simulink model "Quadrotor_Model3D_2018a"  (R2018a)
settings: Solver=VariableStepAuto  StartTime=0.0  StopTime=300  RelTol=1e-3
settings Model: Creator=Slu03  LastModifiedBy=Charles
settings DebuggingCC: LibraryContextMissingDiagnostic=warning
settings SFSimCC: SimUseLocalCustomCode=on
settings RTWCC: RTWUseLocalCustomCode=on

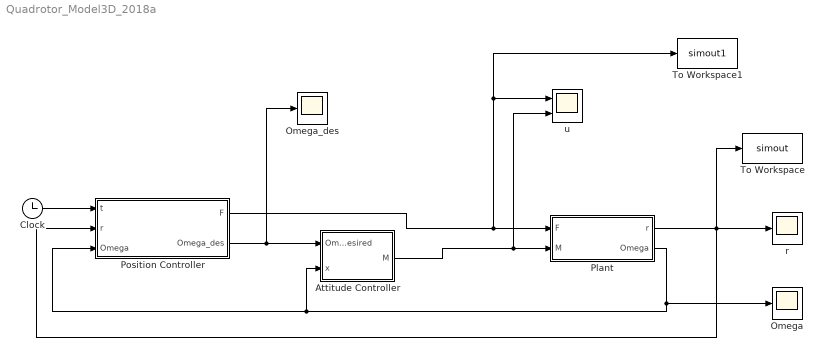
== system Quadrotor_Model3D_2018a ==
  Attitude Controller : MATLAB Function  TreatAsAtomicUnit=on
  Clock : Clock
  Omega : Scope
  Omega_des : Scope
  Plant : Subsystem
  Position Controller : MATLAB Function  TreatAsAtomicUnit=on
  To Workspace : ToWorkspace  VariableName=simout  SaveFormat=Timeseries  SampleTime=-1
  To Workspace1 : ToWorkspace  VariableName=simout1  SaveFormat=Timeseries  SampleTime=-1
  r : Scope
  u : Scope  NumInputPorts=2
  wires:
  Plant/1(r) -> r/1, Position Controller/2(r), To Workspace/1
  Clock/1 -> Position Controller/1(t)
  Position Controller/2(Omega_des) -> Omega_des/1, Attitude Controller/1(Omega_desired)
  Attitude Controller/1(M) -> u/2, Plant/2(M)
  Position Controller/1(F) -> To Workspace1/1, u/1, Plant/1(F)
  Plant/2(Omega) -> Omega/1, Position Controller/3(Omega), Attitude Controller/2(x)

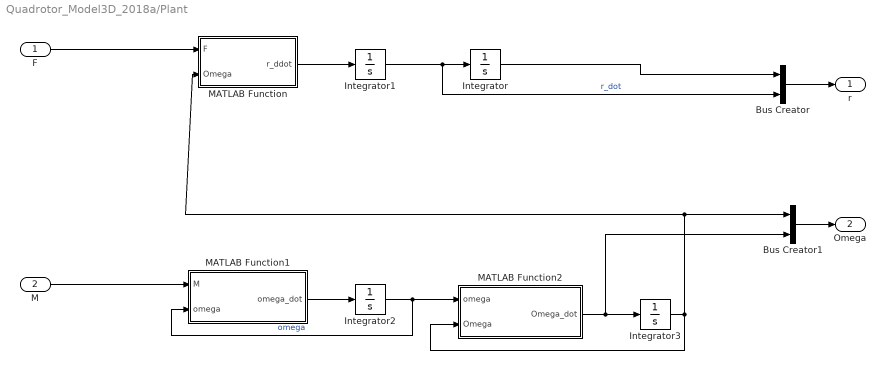
== system Quadrotor_Model3D_2018a/Plant ==
  F : Inport
  M : Inport  Port=2
  Bus Creator : BusCreator  Inputs=2
  Bus Creator1 : BusCreator  Inputs=2
  Integrator : Integrator  InitialCondition=[2,2,0]
  Integrator1 : Integrator
  Integrator2 : Integrator
  Integrator3 : Integrator
  MATLAB Function : MATLAB Function  TreatAsAtomicUnit=on
  MATLAB Function1 : MATLAB Function  TreatAsAtomicUnit=on
  MATLAB Function2 : MATLAB Function  TreatAsAtomicUnit=on
  r : Outport
  Omega : Outport  Port=2
  wires:
  Integrator1/1 -> Bus Creator/2, Integrator/1  "r_dot"
  MATLAB Function/1(r_ddot) -> Integrator1/1
  Integrator2/1 -> MATLAB Function1/2(omega), MATLAB Function2/1(omega)  "omega"
  MATLAB Function1/1(omega_dot) -> Integrator2/1
  MATLAB Function2/1(Omega_dot) -> Bus Creator1/2, Integrator3/1
  Integrator3/1 -> MATLAB Function2/2(Omega), Bus Creator1/1, MATLAB Function/2(Omega)
  F/1 -> MATLAB Function/1(F)
  M/1 -> MATLAB Function1/1(M)
  Bus Creator/1 -> r/1
  Integrator/1 -> Bus Creator/1
  Bus Creator1/1 -> Omega/1

== matlab function Quadrotor_Model3D_2018a/Attitude Controller ==
  data: Omega_desired input; M output; x input
function M = fcn(Omega_desired,x)
kdphi = 20;
kpphi = 100;
kdtheta = 20;
kptheta = 100;
kdpsi = 8;
kppsi = 16;
kd = [kdphi,0,0;0,kdtheta,0;0,0,kdpsi];
kp = [kpphi,0,0;0,kptheta,0;0,0,kppsi];
I = 10^(-5)*[1.43 0 0; 0 1.43 0;0 0 2.89];

Omega_dot = x(4:6);
Omega = x(1:3);
phi = Omega(1);
theta = Omega(2);
psi = Omega(3);

W_inv = [1, 0 ,-sin(theta);0 ,cos(phi),cos(theta)*sin(phi) ; 0 ,-sin(phi),cos(theta)*cos(phi)];
omega = W_inv*Omega_dot;
omega_bracket = [0,-omega(3),omega(2);omega(3),0,-omega(1);-omega(2),omega(1),0];
omega_dot = omega_bracket*I*omega;

M = I*W_inv*(kd*(-Omega_dot)+kp*(Omega_desired-Omega))+omega_dot;

== matlab function Quadrotor_Model3D_2018a/Plant/MATLAB Function ==
  data: F input size=1; Omega input size=3; r_ddot output size=3
function r_ddot = fcn(F,Omega)
g = [0;0;9.8];
m = 0.03;
phi = Omega(1);
theta = Omega(2);
psi = Omega(3);
Rx = [1,0,0; 0,cos(phi),-sin(phi);0,sin(phi),cos(phi)];
Ry = [cos(theta),0,sin(theta);0,1,0;-sin(theta),0,cos(theta)];
Rz = [cos(psi),-sin(psi),0;sin(psi),cos(psi),0;0,0,1];
R = Rz*Ry*Rx;
u = [0;0;F/m];
r_ddot = R*u-g;

== matlab function Quadrotor_Model3D_2018a/Position Controller ==
  data: t input; r input size=6; F output; Omega_des output size=3; Omega input size=6
function [F,Omega_des] = fcn(t,r,Omega)
% r = x y z x_dot y_dot z_dot

m = 0.03;
g = 9.8;
kdx = 2;
kpx = 1;
kdy = 2;
kpy = 1;
kdz = 2;
kpz = 1;

y0 = 2;
x0 = 2;
yh = 5;
xh = 6;
zh = 10;
zt = 8;
psi0 = pi/4;
psih = pi/3;

t1 = 50;
t2 = 100;
T = 100;
t3 = 300;

if t<t1
    x = x0;
    x_dot = 0;
    y = y0;
    y_dot = 0;
    z = zt/t1*t;
    z_dot = zt/t1;
    psi = psi0;
elseif t<t2
    x = x0+(xh-x0)/(t2-t1)*(t-t1);
    x_dot = (xh-x0)/(t2-t1);
    y = y0+(yh-y0)/(t2-t1)*(t-t1);
    y_dot = (yh-y0)/(t2-t1);
    z = zt+(zh-zt)/(t2-t1)*(t-t1);
    z_dot = (zh-zt)/(t2-t1);
    psi = psih;
elseif t<t2+T
    x = xh;
    x_dot = 0;
    y = yh;
    y_dot = 0;
    z = zh;
    z_dot = 0;
    psi = psih;
elseif t<t3
    x = xh;
    x_dot = 0;
    y = yh;
    y_dot = 0;
    z = zh/(t3-t2-T)*(t3-t);
    z_dot = -zh/(t3-t2-T);
    psi = psih;
else
    x = xh;
    x_dot = 0;
    y = yh;
    y_dot = 0; 
    z = 0;
    z_dot = 0;
    psi = psih;
end


x_control = kdx*(x_dot-r(4))+kpx*(x-r(1));
y_control = kdy*(y_dot-r(5))+kpy*(y-r(2));
x_control_hat = cos(Omega(3))*x_control+sin(Omega(3))*y_control;
y_control_hat = -sin(Omega(3))*x_control+cos(Omega(3))*y_control;
z_control = kdz*(z_dot-r(6))+kpz*(z-r(3));

F = m*z_control/(cos(Omega(2))*cos(Omega(1)))+m*g;

phi_des = asin(-y_control_hat/g);
theta_des = asin(x_control_hat/(g*cos(Omega(1))));
psi_des = psi;
Omega_des = [phi_des;theta_des;psi_des];

== matlab function Quadrotor_Model3D_2018a/Plant/MATLAB Function1 ==
  data: M input; omega_dot output size=3; omega input size=3
function omega_dot = fcn(M,omega)
I = 10^(-5)*[1.43 0 0; 0 1.43 0;0 0 2.89];
omega_bracket = [0,-omega(3),omega(2);omega(3),0,-omega(1);-omega(2),omega(1),0];
omega_dot = inv(I)*(M-omega_bracket*I*omega);

== matlab function Quadrotor_Model3D_2018a/Plant/MATLAB Function2 ==
  data: omega input; Omega_dot output; Omega input
function Omega_dot = fcn(omega,Omega)
phi = Omega(1);
theta = Omega(2);
psi = Omega(3);
%W = [1 ,-sin(phi)*tan(theta)/((cos(phi))^2-(sin(phi))^2),-cos(phi)*tan(theta)/((cos(phi))^2-(sin(phi))^2);0,cos(phi)/((cos(phi))^2-(sin(phi))^2),sin(phi)/((cos(phi))^2-(sin(phi))^2);0,sin(phi)/(cos(theta)*((cos(phi))^2-(sin(phi))^2)),cos(phi)/(cos(theta)*((cos(phi))^2-(sin(phi))^2))];
W = [1 tan(theta)*sin(phi) tan(theta)*cos(phi);0,cos(phi),-sin(phi);0,sin(phi)/cos(theta), cos(phi)/cos(theta)];

Omega_dot = W*omega;
